simulink model "guidageLateral"  (R2020b)
settings: Solver=ode45  StartTime=0.0  StopTime=240  RelTol=1e-3
values from neighbouring files (symbols this model uses):
  DEG2RAD = pi/180.    (= 0.0174532925199)    [main.m]
  g = 9.80665    [main.m]
  gammae = 0*DEG2RAD    (= 0)    [main.m]
  k1 = Vp/(g*nze*tauCap)    [main.m]
  k2 = Vp/(g*nze*tauCap*tauEy)    [main.m]
  k3 = 1/tauPhi    (= 0.333333333333)    [main.m]
  KTS2MS = 1852. / 3600.    (= 0.514444444444)    [main.m]
  NM2M = 1852.    (= 1852)    [main.m]
  phiMax = 30*DEG2RAD    (= 0.523598775598)    [main.m]
  psiW = 90*DEG2RAD    (= 1.57079632679)    [main.m]
  Ve = 180*KTS2MS    (= 92.6)    [main.m]
  W = 1*50*KTS2MS    (= 25.7222222222)    [main.m]
libraries: simulink x1
settings Model: Creator=miquelth  LastModifiedBy=florian
settings OptimizationCC: LifeSpan=inf
settings DebuggingCC: AllowSymbolicDim=off  SFExecutionAtInitializationDiag=none  ArithmeticOperatorsInVariantConditions=warning
settings HardwareCC: ProdBitPerSizeT=32  ProdBitPerPtrDiffT=32  ProdWordSize=32  ProdHWDeviceType=Specified
settings SFSimCC: CustomCodeUndefinedFunction=UseInterfaceOnly
settings CodeAppCC: StateflowObjectComments=on

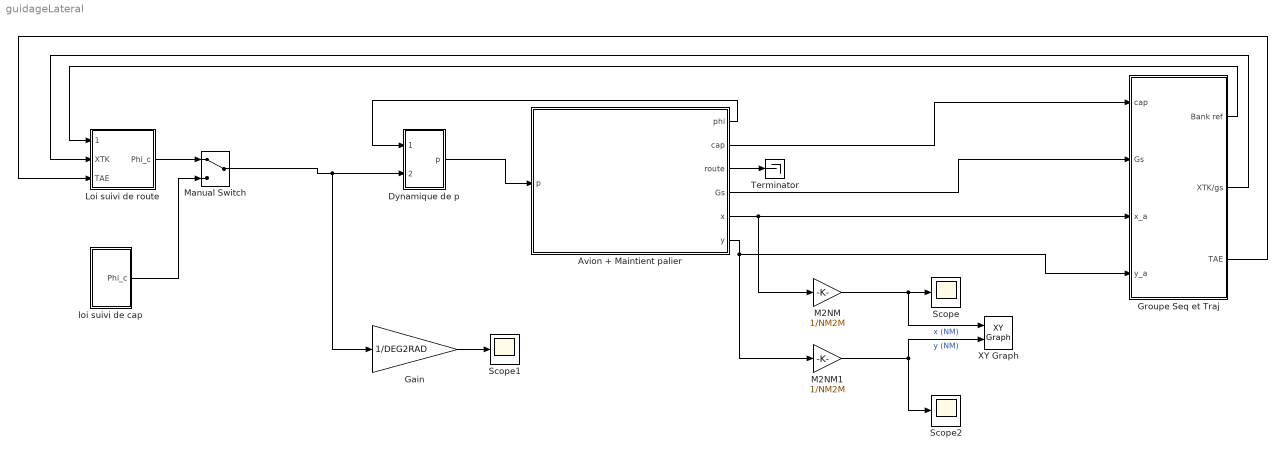
== system guidageLateral ==
  Avion + Maintient palier : Subsystem
  Dynamique de p : Subsystem
  Gain : Gain  Gain=1/DEG2RAD
  Groupe Seq et Traj : Subsystem
  Loi suivi de route : Subsystem
  M2NM : Gain  Gain=1/NM2M
  M2NM1 : Gain  Gain=1/NM2M
  Manual Switch : ManualSwitch
  Scope : Scope
  Scope1 : Scope
  Scope2 : Scope
  Terminator : Terminator
  XY Graph : simulink/Sinks/XY Graph  xmin=-10  xmax=20  ymin=-20  ymax=20  st=-1
  loi suivi de cap : Subsystem
  wires:
  M2NM/1 -> Scope/1, XY Graph/1  "x (NM)"
  M2NM1/1 -> Scope2/1, XY Graph/2  "y (NM)"
  Avion + Maintient palier/3(route) -> Terminator/1
  Avion + Maintient palier/1(phi) -> Dynamique de p/1(phi_a)
  Dynamique de p/1(p) -> Avion + Maintient palier/1(p)
  Gain/1 -> Scope1/1
  Avion + Maintient palier/6(y) -> Groupe Seq et Traj/4(y_a), M2NM1/1
  Avion + Maintient palier/5(x) -> M2NM/1, Groupe Seq et Traj/3(x_a)
  Avion + Maintient palier/2(cap) -> Groupe Seq et Traj/1(cap)
  Avion + Maintient palier/4(Gs) -> Groupe Seq et Traj/2(Gs)
  Groupe Seq et Traj/2(XTK/gs) -> Loi suivi de route/2(XTK)
  Groupe Seq et Traj/3(TAE) -> Loi suivi de route/3(TAE)
  Groupe Seq et Traj/1(Bank ref) -> Loi suivi de route/1(bank angle ref)
  Loi suivi de route/1(Phi_c) -> Manual Switch/1
  Manual Switch/1 -> Gain/1, Dynamique de p/2(phi_c)
  loi suivi de cap/1(Phi_c) -> Manual Switch/2

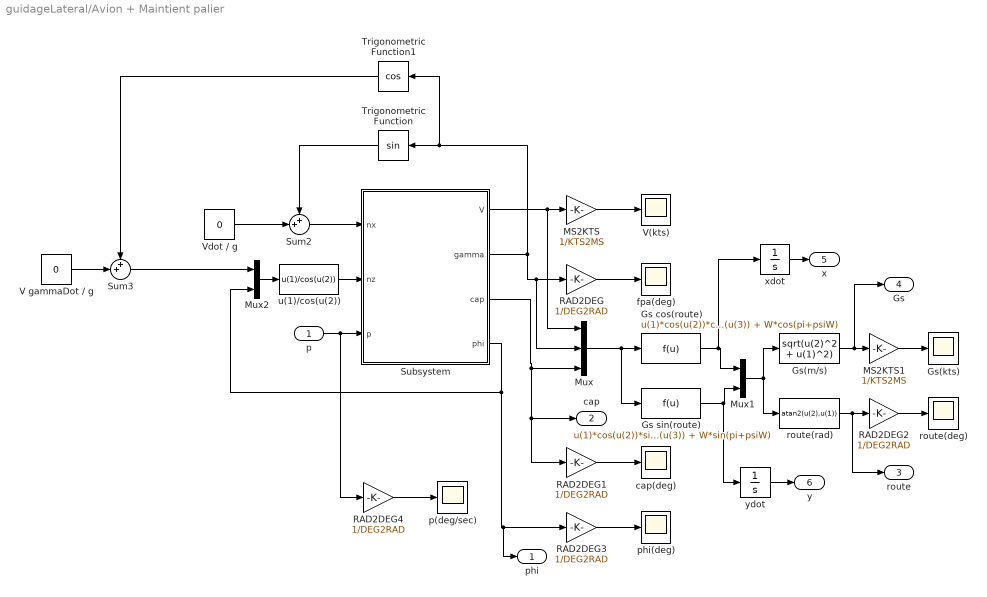
== system guidageLateral/Avion + Maintient palier ==
  p : Inport
  Gs cos(route) : Fcn  Expr=u(1)*cos(u(2))*cos(u(3)) + W*cos(pi+psiW)
  Gs sin(route) : Fcn  Expr=u(1)*cos(u(2))*sin(u(3)) + W*sin(pi+psiW)
  Gs(kts) : Scope
  Gs(m/s) : Fcn  Expr=sqrt(u(2)^2 + u(1)^2)
  MS2KTS : Gain  Gain=1/KTS2MS
  MS2KTS1 : Gain  Gain=1/KTS2MS
  Mux : Mux  Inputs=3
  Mux1 : Mux  Inputs=2
  Mux2 : Mux  Inputs=2
  RAD2DEG{,1..4} (5 alike) : Gain  Gain=1/DEG2RAD
  Subsystem : Subsystem
  Sum2 : Sum  Inputs=++|
  Sum3 : Sum  Inputs=++|
  Trigonometric Function : Trigonometry
  Trigonometric Function1 : Trigonometry  Operator=cos
  V gammaDot / g : Constant  Value=0
  V(kts) : Scope
  Vdot / g : Constant  Value=0
  cap(deg) : Scope
  fpa(deg) : Scope
  p(deg/sec) : Scope
  phi(deg) : Scope
  route(deg) : Scope
  route(rad) : Fcn  Expr=atan2(u(2),u(1))
  u(1)/cos(u(2)) : Fcn  Expr=u(1)/cos(u(2))
  xdot : Integrator
  ydot : Integrator
  phi : Outport
  cap : Outport  Port=2
  route : Outport  Port=3
  Gs : Outport  Port=4
  x : Outport  Port=5
  y : Outport  Port=6
  wires:
  Subsystem/3(cap) -> cap/1, RAD2DEG1/1, Mux/3
  Subsystem/1(V) -> Mux/1, MS2KTS/1
  Subsystem/2(gamma) -> Mux/2, RAD2DEG/1, Trigonometric Function1/1, Trigonometric Function/1
  MS2KTS/1 -> V(kts)/1
  RAD2DEG/1 -> fpa(deg)/1
  Mux/1 -> Gs sin(route)/1, Gs cos(route)/1
  RAD2DEG1/1 -> cap(deg)/1
  Gs cos(route)/1 -> xdot/1, Mux1/1
  Gs sin(route)/1 -> ydot/1, Mux1/2
  Mux1/1 -> route(rad)/1, Gs(m/s)/1
  Gs(m/s)/1 -> Gs/1, MS2KTS1/1
  MS2KTS1/1 -> Gs(kts)/1
  route(rad)/1 -> route/1, RAD2DEG2/1
  RAD2DEG2/1 -> route(deg)/1
  Subsystem/4(phi) -> Mux2/2, phi/1, RAD2DEG3/1
  RAD2DEG3/1 -> phi(deg)/1
  Vdot / g/1 -> Sum2/2
  Trigonometric Function/1 -> Sum2/1
  Sum2/1 -> Subsystem/1(nx)
  V gammaDot / g/1 -> Sum3/2
  Trigonometric Function1/1 -> Sum3/1
  Mux2/1 -> u(1)/cos(u(2))/1
  u(1)/cos(u(2))/1 -> Subsystem/2(nz)
  Sum3/1 -> Mux2/1
  RAD2DEG4/1 -> p(deg/sec)/1
  xdot/1 -> x/1
  ydot/1 -> y/1
  p/1 -> RAD2DEG4/1, Subsystem/3(p)

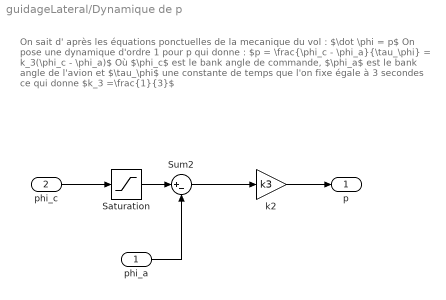
== system guidageLateral/Dynamique de p ==
  note: On sait d' après les équations ponctuelles de la mecanique du vol : $\dot \phi = p$
      | On pose une dynamique d'ordre 1 pour p qui donne : $p = \frac{\phi_c - \phi_a}{\tau_\phi} = k_3(\phi_c - \phi_a)$
      | Où $\phi_c$ est le bank angle de commande, $\phi_a$ est le bank angle de l'avion
      | et $\tau_\phi$ une constante de temps que l'on fixe égale à 3 secondes ce qui donne $k_3 =\frac{1}{3}$
  phi_a : Inport
  phi_c : Inport  Port=2
  Saturation : Saturate  UpperLimit=phiMax  LowerLimit=-phiMax
  Sum2 : Sum  Inputs=|+-
  k2 : Gain  Gain=k3
  p : Outport
  wires:
  Sum2/1 -> k2/1
  k2/1 -> p/1
  Saturation/1 -> Sum2/1
  phi_c/1 -> Saturation/1
  phi_a/1 -> Sum2/2

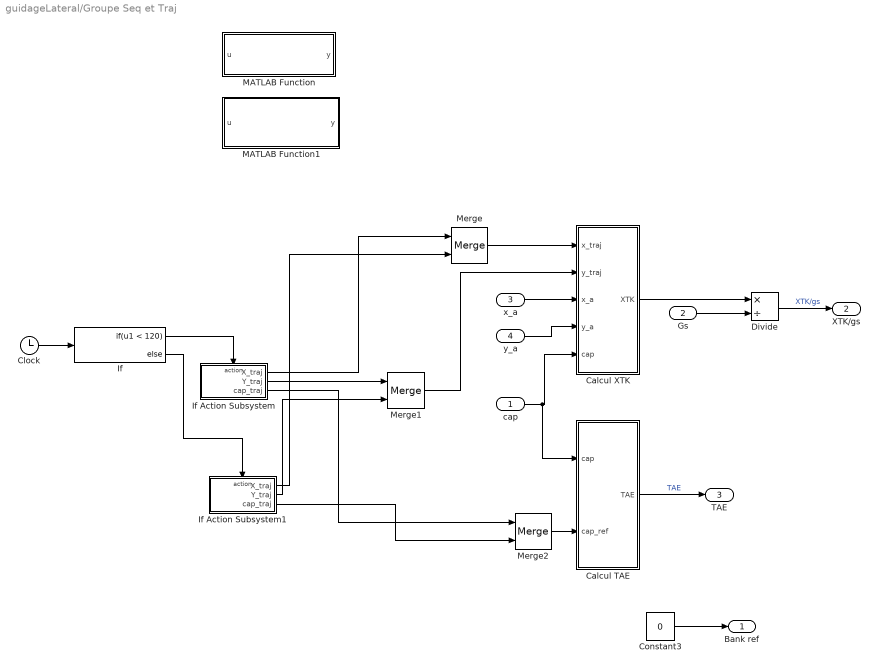
== system guidageLateral/Groupe Seq et Traj ==
  cap : Inport
  Gs : Inport  Port=2
  x_a : Inport  Port=3
  y_a : Inport  Port=4
  Calcul TAE : MATLAB Function  TreatAsAtomicUnit=on
  Calcul XTK : MATLAB Function  TreatAsAtomicUnit=on
  Clock : Clock
  Constant3 : Constant  Value=0
  Divide : Product  Inputs=*/
  If : If  IfExpression=u1 < 120
  If Action Subsystem : Subsystem  TreatAsAtomicUnit=on
  If Action Subsystem1 : Subsystem  TreatAsAtomicUnit=on
  MATLAB Function : MATLAB Function  TreatAsAtomicUnit=on
  MATLAB Function1 : MATLAB Function  TreatAsAtomicUnit=on
  Merge : Merge
  Merge1 : Merge
  Merge2 : Merge
  Bank ref : Outport
  XTK/gs : Outport  Port=2
  TAE : Outport  Port=3
  wires:
  x_a/1 -> Calcul XTK/3(x_a)
  Divide/1 -> XTK/gs/1  "XTK/gs"
  Gs/1 -> Divide/2
  Calcul TAE/1(TAE) -> TAE/1  "TAE"
  Calcul XTK/1(XTK) -> Divide/1
  y_a/1 -> Calcul XTK/4(y_a)
  Merge/1 -> Calcul XTK/1(x_traj)
  Merge2/1 -> Calcul TAE/2(cap_ref)
  cap/1 -> Calcul TAE/1(cap), Calcul XTK/5(cap)
  Merge1/1 -> Calcul XTK/2(y_traj)
  Constant3/1 -> Bank ref/1
  Clock/1 -> If/1
  If/1 -> If Action Subsystem/Action
  If/2 -> If Action Subsystem1/Action
  If Action Subsystem/1(X_traj) -> Merge/1
  If Action Subsystem1/1(X_traj) -> Merge/2
  If Action Subsystem/2(Y_traj) -> Merge1/1
  If Action Subsystem1/2(Y_traj) -> Merge1/2
  If Action Subsystem/3(cap_traj) -> Merge2/1
  If Action Subsystem1/3(cap_traj) -> Merge2/2

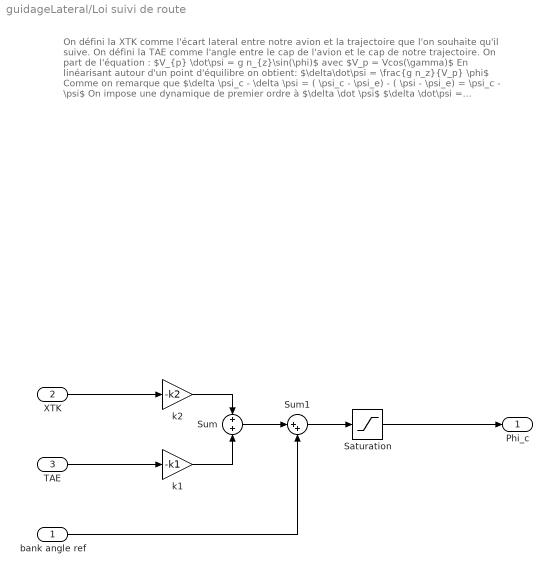
== system guidageLateral/Loi suivi de route ==
  note: On défini la XTK comme l'écart lateral entre notre avion et la trajectoire que l'on souhaite qu'il suive.
      | On défini la TAE comme l'angle entre le cap de l'avion et le cap de notre trajectoire.
      | On part de l'équation :
      | $V_{p} \dot\psi = g n_{z}\sin(\phi)$ avec $V_p = Vcos(\gamma)$
      | En linéarisant autour d'un point d'équilibre on obtient:
      | $\delta\dot\psi = \frac{g n_z}{V_p} \phi$
      | Comme on remarque que $\delta \psi_c - \delta \psi = ( \psi_c - \psi_e) - ( \psi - \psi_e) = \psi_c - \psi$
      | On impose une dynamique de premier ordre à $\delta \dot \psi$
      | $\delta \dot\psi = \frac{\delta\psi_c - \delta\psi}{\tau_\psi} = \frac{\psi_c - \psi}{\tau_\psi}$
      | avec $\tau_\psi$ une contante de temps.
      | Il vient donc en assimilant $\phi \approx \phi_c$ :
      | $\delta\dot\psi = \frac{g n_z}{V_p} \phi \approx \frac{g n_z}{V_p} \phi_c$
      | Ce qui nous donne:
      | $\phi_c = \frac{V_p}{g n_z} \frac{\psi_c - \psi}{\tau_\psi}$
  bank angle ref : Inport
  XTK : Inport  Port=2
  TAE : Inport  Port=3
  Saturation : Saturate  UpperLimit=phiMax  LowerLimit=-phiMax
  Sum : Sum
  Sum1 : Sum  Inputs=|++
  k1 : Gain  Gain=-k1
  k2 : Gain  Gain=-k2
  Phi_c : Outport
  wires:
  k1/1 -> Sum/2
  XTK/1 -> k2/1
  TAE/1 -> k1/1
  k2/1 -> Sum/1
  Sum/1 -> Sum1/1
  bank angle ref/1 -> Sum1/2
  Sum1/1 -> Saturation/1
  Saturation/1 -> Phi_c/1

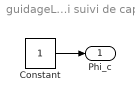
== system guidageLateral/loi suivi de cap ==
  Constant : Constant
  Phi_c : Outport
  wires:
  Constant/1 -> Phi_c/1

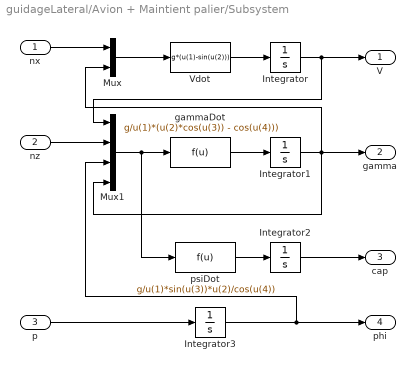
== system guidageLateral/Avion + Maintient palier/Subsystem ==
  nx : Inport
  nz : Inport  Port=2
  p : Inport  Port=3
  Integrator : Integrator  InitialCondition=Ve
  Integrator1 : Integrator  InitialCondition=gammae
  Integrator2 : Integrator
  Integrator3 : Integrator
  Mux : Mux  Inputs=2
  Mux1 : Mux
  Vdot : Fcn  Expr=g*(u(1)-sin(u(2)))
  gammaDot : Fcn  Expr=g/u(1)*(u(2)*cos(u(3)) - cos(u(4)))
  psiDot : Fcn  Expr=g/u(1)*sin(u(3))*u(2)/cos(u(4))
  V : Outport
  gamma : Outport  Port=2
  cap : Outport  Port=3
  phi : Outport  Port=4
  wires:
  Mux/1 -> Vdot/1
  nz/1 -> Mux1/2
  Vdot/1 -> Integrator/1
  Integrator/1 -> V/1, Mux1/1
  Mux1/1 -> psiDot/1, gammaDot/1
  gammaDot/1 -> Integrator1/1
  Integrator1/1 -> gamma/1, Mux1/4, Mux/2
  psiDot/1 -> Integrator2/1
  Integrator2/1 -> cap/1
  nx/1 -> Mux/1
  p/1 -> Integrator3/1
  Integrator3/1 -> phi/1, Mux1/3

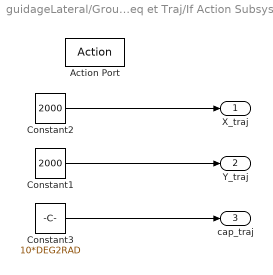
== system guidageLateral/Groupe Seq et Traj/If Action Subsystem ==
  Action Port : ActionPort  ActionPortLabel=if(u1 < 120)
  Constant1 : Constant  Value=2000
  Constant2 : Constant  Value=2000
  Constant3 : Constant  Value=10*DEG2RAD
  X_traj : Outport
  Y_traj : Outport  Port=2
  cap_traj : Outport  Port=3
  wires:
  Constant2/1 -> X_traj/1
  Constant1/1 -> Y_traj/1
  Constant3/1 -> cap_traj/1

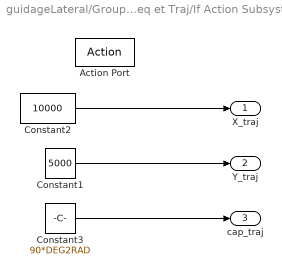
== system guidageLateral/Groupe Seq et Traj/If Action Subsystem1 ==
  Action Port : ActionPort  ActionPortLabel=else
  Constant1 : Constant  Value=5000
  Constant2 : Constant  Value=10000
  Constant3 : Constant  Value=90*DEG2RAD
  X_traj : Outport
  Y_traj : Outport  Port=2
  cap_traj : Outport  Port=3
  wires:
  Constant2/1 -> X_traj/1
  Constant1/1 -> Y_traj/1
  Constant3/1 -> cap_traj/1

== matlab function guidageLateral/Groupe Seq et Traj/MATLAB Function1 ==
  data: u input; y output
function y = limitPlusPiMoinsPiSat(u)
    y = u;
    while y > pi
        y = y-2*pi;
    end
    while y < -pi
        y = y+2*pi;
    end
    %limitation de l'angle de convergence
    DEG2RAD = pi/180;
    deltaDirMax = 45*DEG2RAD; 
    if y > deltaDirMax
        y = deltaDirMax;
    elseif y < -deltaDirMax
        y = -deltaDirMax;
    end
end

== matlab function guidageLateral/Groupe Seq et Traj/MATLAB Function ==
  data: u input; y output
function y = limitPlusPiMoinsPi(u)
    y = u;
    while y > pi
        y = y-2*pi;
    end
    while y < -pi
        y = y+2*pi;
    end
end

== matlab function guidageLateral/Groupe Seq et Traj/Calcul XTK ==
  data: x_traj input; XTK output; y_traj input; x_a input; y_a input; cap input
function XTK = fcn(x_traj, y_traj, x_a, y_a, cap)
    XTK = -sin(cap)*(x_traj-x_a) + cos(cap)*(y_traj-y_a);
end

== matlab function guidageLateral/Groupe Seq et Traj/Calcul TAE ==
  data: cap input; cap_ref input; TAE output
function TAE = fcn(cap, cap_ref)
    TAE = cap-cap_ref;
end
